simulink model "edfh_sim"  (R2022b)
settings: Solver=VariableStepAuto  StartTime=0.0  StopTime=20  RelTol=1e-3
values from neighbouring files (symbols this model uses):
  g = 9.807    [nonlin_dynamics.m]    (also in nonlinear_dynamics_edfh.m)
  G_hov = [ 0 0 0 0 0 0 1 0 ]    [nonlinear_dynamics_edfh.m]
  G_pos = [ 1 0 0 0 ... (first row only)    [nonlinear_dynamics_edfh.m]
  K_pos = lqr(sys_hor, Q_pos, R_pos)    [nonlinear_dynamics_edfh.m]
  K_red = lqr(sys_red, Q_red, R_red)    [nonlinear_dynamics_edfh.m]
  m = 2.300    (= 2.3)    [nonlin_dynamics.m]    (also in nonlinear_dynamics_edfh.m)
libraries: mcbcontrolslib x4, simulink x2
settings Model: Creator=mak  LastModifiedBy=mak

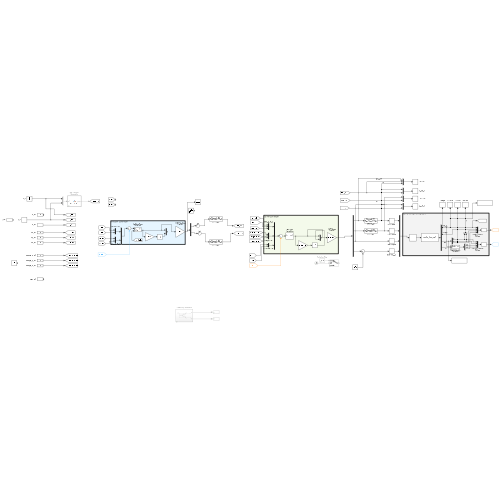
[thumbnail: Simulink's stored preview of the top-level diagram]
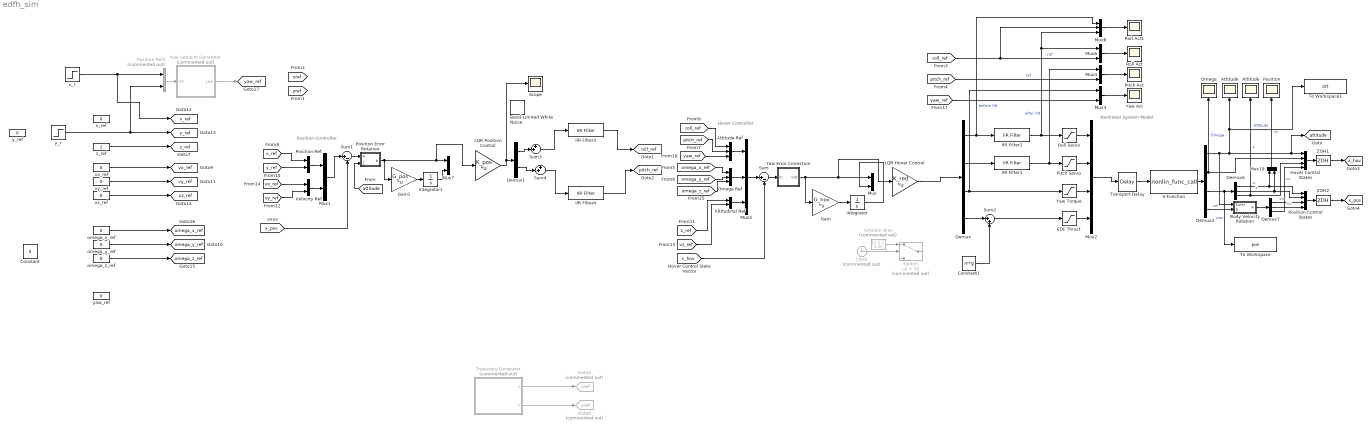
== system edfh_sim ==
  note: Hover Controller
  note: Nonlinear System Model
  note: Position Controller
  Actuator Bias : Constant  Commented=on  Value=[1 1 1 1 0]
  Altitude : Scope
  Altitudinal Ref : Mux  Inputs=2
  Attitude : Scope
  Attitude Ref : Mux  Inputs=3
  Band-Limited White Noise : simulink/Sources/Band-Limited White Noise  Cov=[0.0001]  Ts=0.005  seed=[23341]
  Body Velocity Rotation : Subsystem
  Clock : Clock  Commented=on
  Constant : Constant  Value=0
  Constant1 : Constant  Value=m*g
  Demux : Demux
  Demux1 : Demux  Outputs=2
  Demux2 : Demux
  Demux6 : Demux  Outputs=3
  Demux7 : Demux  Outputs=3
  EDF Thrust : Saturate  UpperLimit=31  LowerLimit=0
  Gain : Gain  Gain=G_hov  Multiplication=Matrix(K*u)
  Gain1 : Gain  Gain=G_pos  Multiplication=Matrix(K*u)
  Goto5 : Goto  Commented=on  GotoTag=xref  TagVisibility=global
  Goto6 : Goto  Commented=on  GotoTag=yref  TagVisibility=global
  Hover Control States : Mux
  IIR Filter1 : mcbcontrolslib/IIR Filter  VariantControl=Low Pass Filter  VariantSelect=Low-pass  Filter_constant=0.75  advancedSettings=off  Ts=50e-6  cutOff_freq=9549.2966
      settings: LibrarySourceBlock=mcblib/Signal Management/IIR Filter
  IIR Filter2 : mcbcontrolslib/IIR Filter  VariantControl=Low Pass Filter  VariantSelect=Low-pass  Filter_constant=0.75  advancedSettings=off  Ts=50e-6  cutOff_freq=9549.2966
      settings: LibrarySourceBlock=mcblib/Signal Management/IIR Filter
  IIR Filter3 : mcbcontrolslib/IIR Filter  VariantControl=Low Pass Filter  VariantSelect=Low-pass  Filter_constant=0.55  advancedSettings=off  Ts=50e-6  cutOff_freq=3890.4542
      settings: LibrarySourceBlock=mcblib/Signal Management/IIR Filter
  IIR Filter4 : mcbcontrolslib/IIR Filter  VariantControl=Low Pass Filter  VariantSelect=Low-pass  Filter_constant=0.55  advancedSettings=off  Ts=50e-6  cutOff_freq=3890.4542
      settings: LibrarySourceBlock=mcblib/Signal Management/IIR Filter
  Integrator : Integrator  LimitOutput=on  UpperSaturationLimit=1  LowerSaturationLimit=0
  Integrator1 : Integrator  LimitOutput=on  UpperSaturationLimit=0.4  LowerSaturationLimit=-0.4
  LQR Hover Control : Gain  Gain=K_red  Multiplication=Matrix(K*u)
  LQR Position Control : Gain  Gain=K_pos  Multiplication=Matrix(K*u)
  Mux{,1,3..4,6..7,10} (7 alike) : Mux  Inputs=2
  Mux2 : Mux
  Mux5 : Mux  Inputs=3
  Mux8 : Mux  Inputs=3
  Omega : Scope
  Omega Ref : Mux  Inputs=3
  Pitch Act : Scope
  Pitch Servo : Saturate  UpperLimit=0.24  LowerLimit=-0.24
  Position : Scope
  Position Control States : Mux
  Position Error Rotation : Subsystem
  Position Ref : Mux  Inputs=2
  Position Ref2 : Mux  Commented=on  Inputs=2
  Roll Act : Scope
  Roll Act1 : Scope
  "Roll Servo " : Saturate  UpperLimit=0.24  LowerLimit=-0.24
  S-Function : S-Function  FunctionName=nonlin_func_call  SFunctionDeploymentMode=off  EnableBusSupport=off
  Scope : Scope
  Sum : Sum  Inputs=|+-
  Sum1 : Sum  Inputs=|+-
  Sum2 : Sum  Inputs=|++
  Sum3 : Sum  Inputs=++|
  Sum4 : Sum  Inputs=++|
  Switch : Switch  Commented=on  Criteria=u2 > Threshold  Threshold=20  SaturateOnIntegerOverflow=off  InputSameDT=off
  To Workspace : ToWorkspace  VariableName=pos  SaveFormat=Timeseries  SampleTime=-1
  To Workspace1 : ToWorkspace  VariableName=att  SaveFormat=Timeseries  SampleTime=-1
  Trajectory Generator : Subsystem  Commented=on
  Transport Delay : TransportDelay  DelayTime=.001
  Velocity Ref : Mux  Inputs=2
  Yaw Act : Scope
  Yaw Error Correction : Subsystem
  Yaw Setpoint Generator : MATLAB Function  Commented=on  TreatAsAtomicUnit=on
  Yaw Torque : Saturate  UpperLimit=2  LowerLimit=0
  ZOH1 : ZeroOrderHold  SampleTime=0.005
  ZOH2 : ZeroOrderHold  SampleTime=0.005
  omega_x_ref : Constant  Value=0
  omega_y_ref : Constant  Value=0
  omega_z_ref : Constant  Value=0
  vx_ref : Constant  Value=0
  vy_ref : Constant  Value=0
  vz_ref : Constant  Value=0
  x_r : Step  Time=4  After=3  SampleTime=0
  x_ref : Constant  Value=0
  y_r : Step  Time=10  After=2  SampleTime=0
  y_ref : Constant  Value=0
  yaw_ref : Constant  Value=0
  z_ref : Constant
  tag scope: attitude=global, omega_x_ref=global, omega_y_ref=global, omega_z_ref=global, pitch_ref=global, roll_ref=global, vx_ref=global, vy_ref=global, vz_ref=global, x_hov=global, x_pos=global, x_ref=global, y_ref=global, yaw_ref=global, z_ref=global
  wires:
  Integrator/1 -> Mux/2
  Sum/1 -> Yaw Error Correction/1(in)
  Demux1/1 -> Sum3/2
  [x_pos] -> Sum1/2
  Demux7/3 -> Hover Control States/4  "vz"
  ZOH2/1 -> [x_pos]
  Mux1/1 -> Sum1/1
  Hover Control States/1 -> ZOH1/1
  Demux7/1 -> Position Control States/3  "vx"
  Gain/1 -> Integrator/1
  Demux6/1 -> Position Control States/1, Mux10/1  "x"
  Gain1/1 -> Integrator1/1
  Demux2/2 -> Hover Control States/2, Omega/1  "Omega"
  Demux6/3 -> Hover Control States/3, Altitude/1  "z"
  Altitudinal Ref/1 -> Mux5/3
  Trajectory Generator/2(y) -> Goto6/1
  ZOH1/1 -> [x_hov]
  LQR Position Control/1 -> Scope/1, Demux1/1
  Demux6/2 -> Mux10/2, Position Control States/2  "y"
  S-Function/1 -> Demux2/1
  Demux1/2 -> Sum4/2
  Velocity Ref/1 -> Mux1/2
  Actuator Bias/1 -> Switch/1
  Mux10/1 -> Position/1  "xy"
  [pitch_ref] -> Attitude Ref/2
  Demux7/2 -> Position Control States/4  "vy"
  Attitude Ref/1 -> Mux5/1
  Omega Ref/1 -> Mux5/2
  Position Error Rotation/1(b) -> LQR Position Control/1, Mux7/1, Gain1/1
  Clock/1 -> Switch/2
  Demux2/3 -> To Workspace/1, Demux6/1  "pos"
  Body Velocity Rotation/1(w) -> Demux7/1
  [z_ref] -> Altitudinal Ref/1
  [attitude] -> Position Error Rotation/2(Euler)
  Sum1/1 -> Position Error Rotation/1(w)
  x_r/1 -> [x_ref], Position Ref2/1
  Position Ref2/1 -> Yaw Setpoint Generator/1(ref)
  [roll_ref] -> Attitude Ref/1
  Position Ref/1 -> Mux1/1
  Mux5/1 -> Sum/1
  [x_hov] -> Sum/2
  Demux2/1 -> To Workspace1/1, Attitude/1, [attitude], Hover Control States/1, Body Velocity Rotation/1(Euler)  "Attitude"
  Integrator1/1 -> Mux7/2
  Trajectory Generator/1(x) -> Goto5/1
  Position Control States/1 -> ZOH2/1
  Demux2/4 -> Body Velocity Rotation/2(b)  "vel"
  Yaw Error Correction/1(out) -> Gain/1, LQR Hover Control/1, Mux/1
  [vz_ref] -> Altitudinal Ref/2
  [x_ref] -> Position Ref/1
  [y_ref] -> Position Ref/2
  [vx_ref] -> Velocity Ref/1
  [vy_ref] -> Velocity Ref/2
  [omega_x_ref] -> Omega Ref/1
  [omega_y_ref] -> Omega Ref/2
  [omega_z_ref] -> Omega Ref/3
  [yaw_ref] -> Attitude Ref/3
  z_ref/1 -> [z_ref]
  vx_ref/1 -> [vx_ref]
  vy_ref/1 -> [vy_ref]
  vz_ref/1 -> [vz_ref]
  omega_y_ref/1 -> [omega_y_ref]
  omega_z_ref/1 -> [omega_z_ref]
  Mux2/1 -> Transport Delay/1
  Demux/3 -> Yaw Torque/1, Mux3/1
  "Roll Servo "/1 -> Mux2/1
  Pitch Servo/1 -> Mux2/2
  Yaw Torque/1 -> Mux2/3
  EDF Thrust/1 -> Mux2/4
  omega_x_ref/1 -> [omega_x_ref]
  Constant1/1 -> Sum2/2
  Demux/4 -> Sum2/1
  Sum2/1 -> EDF Thrust/1
  Mux6/1 -> Roll Act/1
  Mux4/1 -> Pitch Act/1
  Mux3/1 -> Yaw Act/1
  [yaw_ref] -> Mux3/2
  [pitch_ref] -> Mux4/2  "ref"
  [roll_ref] -> Mux8/2, Mux6/2  "ref"
  Yaw Setpoint Generator/1(yaw) -> [yaw_ref]
  Demux/1 -> IIR Filter2/1, Mux8/1  "before filt"
  Sum3/1 -> IIR Filter3/1
  Sum4/1 -> IIR Filter4/1
  Demux/2 -> IIR Filter1/1
  Mux8/1 -> Roll Act1/1
  IIR Filter1/1 -> Mux4/1, Pitch Servo/1
  IIR Filter2/1 -> Mux6/1, Mux8/3, "Roll Servo "/1  "after filt"
  IIR Filter3/1 -> [roll_ref]
  IIR Filter4/1 -> [pitch_ref]
  Transport Delay/1 -> S-Function/1
  LQR Hover Control/1 -> Demux/1
  y_r/1 -> Position Ref2/2, [y_ref]

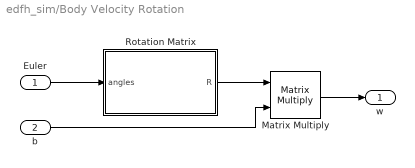
== system edfh_sim/Body Velocity Rotation ==
  Euler : Inport
  b : Inport  Port=2
  Matrix Multiply : Product  Multiplication=Matrix(*)
  Rotation Matrix : MATLAB Function  TreatAsAtomicUnit=on
  w : Outport
  wires:
  Rotation Matrix/1(R) -> Matrix Multiply/1
  Euler/1 -> Rotation Matrix/1(angles)
  b/1 -> Matrix Multiply/2
  Matrix Multiply/1 -> w/1

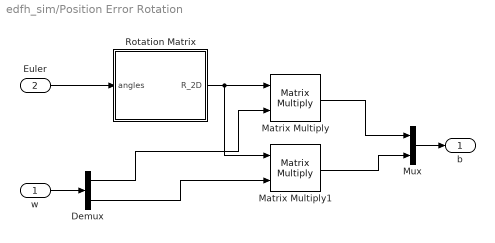
== system edfh_sim/Position Error Rotation ==
  w : Inport
  Euler : Inport  Port=2
  Demux : Demux  Outputs=2
  Matrix Multiply : Product  Multiplication=Matrix(*)
  Matrix Multiply1 : Product  Multiplication=Matrix(*)
  Mux : Mux  Inputs=2
  Rotation Matrix : MATLAB Function  TreatAsAtomicUnit=on
  b : Outport
  wires:
  Rotation Matrix/1(R_2D) -> Matrix Multiply1/1, Matrix Multiply/1
  Euler/1 -> Rotation Matrix/1(angles)
  Matrix Multiply/1 -> Mux/1
  w/1 -> Demux/1
  Demux/2 -> Matrix Multiply1/2
  Demux/1 -> Matrix Multiply/2
  Matrix Multiply1/1 -> Mux/2
  Mux/1 -> b/1

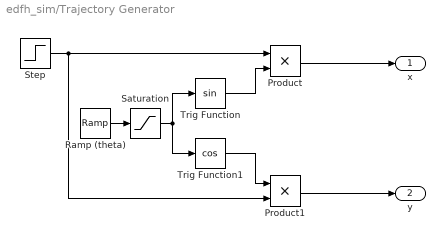
== system edfh_sim/Trajectory Generator ==
  Product : Product  RndMeth=Zero
  Product1 : Product  RndMeth=Zero
  Ramp (theta) : simulink/Sources/Ramp  slope=pi / 20  start=20  InitialOutput=0
  Saturation : Saturate  UpperLimit=2 * pi  LowerLimit=0
  Step : Step  Time=20  SampleTime=0
  Trig Function : Trigonometry
  Trig Function1 : Trigonometry  Operator=cos
  x : Outport
  y : Outport  Port=2
  wires:
  Product/1 -> x/1
  Step/1 -> Product1/2, Product/1
  Ramp (theta)/1 -> Saturation/1
  Trig Function1/1 -> Product1/1
  Saturation/1 -> Trig Function/1, Trig Function1/1
  Trig Function/1 -> Product/2
  Product1/1 -> y/1

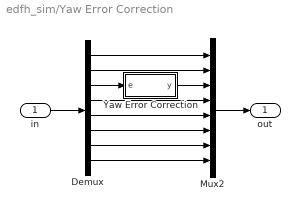
== system edfh_sim/Yaw Error Correction ==
  in : Inport
  Demux : Demux  Outputs=8
  Mux2 : Mux  Inputs=8
  Yaw Error Correction : MATLAB Function  TreatAsAtomicUnit=on
  out : Outport
  wires:
  Demux/8 -> Mux2/8
  Demux/2 -> Mux2/2
  Yaw Error Correction/1(y) -> Mux2/3
  Demux/1 -> Mux2/1
  Demux/3 -> Yaw Error Correction/1(e)
  Demux/7 -> Mux2/7
  Demux/6 -> Mux2/6
  Demux/4 -> Mux2/4
  Demux/5 -> Mux2/5
  Mux2/1 -> out/1
  in/1 -> Demux/1

== matlab function edfh_sim/Yaw Setpoint Generator ==
  settings: updateMethod=DISCRETE
  data: ref input; yaw output size=1
function yaw = yaw_setpoint(ref)

persistent last_ref

if isempty(last_ref)
    last_ref = ref;
end

dx = ref(1) - last_ref(1);
dy = ref(2) - last_ref(2);

last_ref = ref;

yaw = atan2( dy, dx );

== matlab function edfh_sim/Position Error Rotation/Rotation Matrix ==
  data: angles input size=[3 1]; R_2D output size=[2 2]
function R_2D = world_to_body( angles )

    p = 0;
    q = 0;
    u = angles(3);
    
    R_2D = [ cos(q)*cos(u),                         cos(q)*sin(u),                        ;
             cos(u)*sin(p)*sin(q) - cos(p)*sin(u),  cos(p)*cos(u) + sin(p)*sin(q)*sin(u) ];

== matlab function edfh_sim/Yaw Error Correction/Yaw Error Correction ==
  data: e input; y output
function y = fcn(e)
    
    % Correct yaw error
    if( e > pi )
        e = e - 2 * pi;
    end
    
    y = e;
    
end

== matlab function edfh_sim/Body Velocity Rotation/Rotation Matrix ==
  data: angles input size=[3 1]; R output size=[3 3]
function R = body_to_world( angles )

    p = angles(1);
    q = angles(2);
    u = angles(3);
    

    R = [cos(q)*cos(u), sin(p)*sin(q)*cos(u)-cos(p)*sin(u), cos(p)*sin(q)*cos(u)+sin(p)*sin(u) ;
         cos(q)*sin(u), sin(p)*sin(q)*sin(u)+cos(p)*cos(u), cos(p)*sin(q)*sin(u)-sin(p)*cos(u) ;
         -sin(q),       sin(p)*cos(q),                      cos(p)*cos(q)                     ];
